simulink model "LTI_test"  (R2016b)
settings: Solver=VariableStepAuto  StartTime=0.0  StopTime=10.0  RelTol=1e-3
values from neighbouring files (symbols this model uses):
  A = [ -0.2, 0.1, -1 ... (first row only)    [testLTI.m]
  A1 = [0 ,- 0.1 ... (first row only)    [testLTI.m]
  B = [ 2, 2, 3]'    [testLTI.m]
  B1 = [0;1]    [testLTI.m]
  C = [ 1, 0, 0 ... (first row only)    [testLTI.m]
  C1 = [1, 0 ... (first row only)    [testLTI.m]
  D = [ 0,0,0]'    [testLTI.m]
  D1 = [0, 0]'    [testLTI.m]
  x0 = [0 0 0]'    [testLTI.m]
  x1 = [0,1]'    [testLTI.m]
settings Model: Creator=arthus  LastModifiedBy=arthus

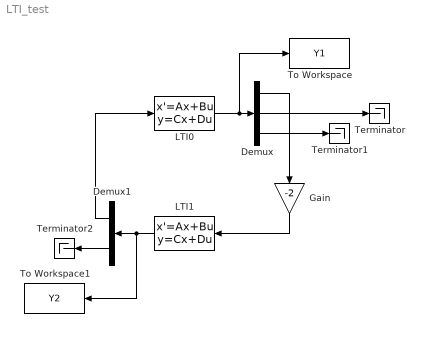
== system LTI_test ==
  Demux : Demux  Outputs=3
  Demux1 : Demux  Outputs=2
  Gain : Gain  Gain=-2
  LTI0 : StateSpace  A=A  B=B  C=C  D=D  X0=x0
  LTI1 : StateSpace  A=A1  B=B1  C=C1  D=D1  X0=x1
  Terminator : Terminator
  Terminator1 : Terminator
  Terminator2 : Terminator
  To Workspace : ToWorkspace  VariableName=Y1  SaveFormat=Timeseries  SampleTime=-1
  To Workspace1 : ToWorkspace  VariableName=Y2  SaveFormat=Timeseries  SampleTime=-1
  wires:
  Gain/1 -> LTI1/1
  LTI0/1 -> To Workspace/1, Demux/1
  Demux/1 -> Gain/1
  Demux/2 -> Terminator/1
  Demux/3 -> Terminator1/1
  Demux1/2 -> Terminator2/1
  LTI1/1 -> To Workspace1/1, Demux1/1
  Demux1/1 -> LTI0/1
